simulink model "Hello_World"  (R2014a)
settings: Solver=FixedStepDiscrete  StartTime=0.0  StopTime=10  FixedStep=0.01  RelTol=1e-3
PostLoadFcn:
  | T = 0.1;
CloseFcn:
  | clear T
settings Model: Creator=The MathWorks Inc.  LastModifiedBy=darenlee
settings OptimizationCC: OptimizeModelRefInitCode=on  LifeSpan=1  MaxStackSize=64
settings DebuggingCC: UnderspecifiedInitializationDetection=Classic
settings HardwareCC: ProdLargestAtomicInteger=Long  ProdLargestAtomicFloat=Double  ProdEndianess=LittleEndian  ProdHWDeviceType=ARM Compatible->ARM Cortex
settings RTWCC: SystemTargetFile=ert.tlc  TemplateMakefile=ert_default_tmf  PostCodeGenCommand=; codertarget.postCodeGenHookCommand(h)  Description=Embedded Coder  GenerateReport=on  ProcessScript=ert_make_rtw_hook  Toolchain=Code Sourcery  IncludeHyperlinkInReport=on  LaunchReport=on  GenerateTraceInfo=on  GenerateTraceReport=on  GenerateTraceReportSl=on  GenerateTraceReportSf=on  GenerateTraceReportEml=on
settings CodeAppCC: IgnoreCustomStorageClasses=off
settings ERTTargetCC: ParMdlRefBuildCompliant=on  CompOptLevelCompliant=on  ConcurrentExecutionCompliant=on  ERTFirstTimeCompliant=on  ModelStepFunctionPrototypeControlCompliant=on  CPPClassGenCompliant=on  ExtMode=on  ExtModeMexArgs='192.168.1.1' 1 17725  InlinedParameterPlacement=Hierarchical

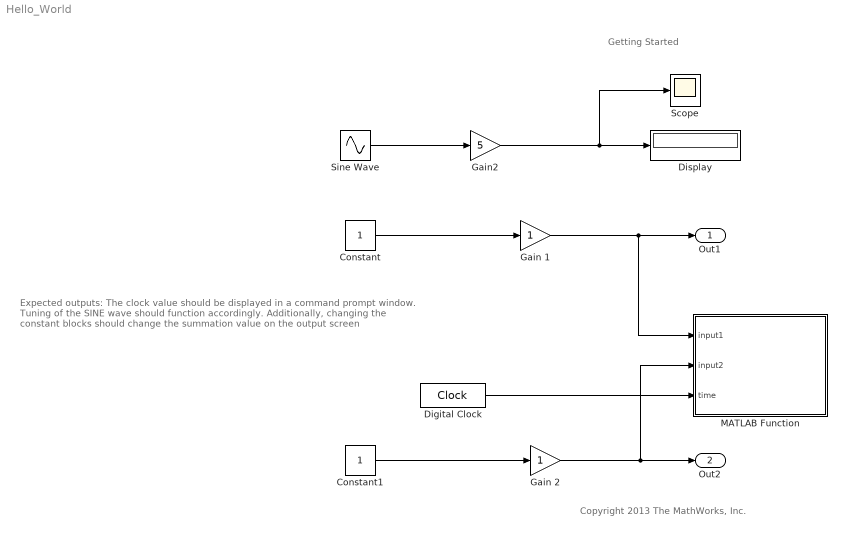
== system Hello_World ==
  note: Expected outputs:
      |
      | The clock value should be displayed in a command prompt window. Tuning
      | of the SINE wave should function accordingly. Additionally, changing the
      | constant blocks should change the summation value on the output screen
  note: Getting Started
  note: Copyright 2013 The MathWorks, Inc.
  Constant : Constant
  Constant1 : Constant
  Digital Clock : DigitalClock  SampleTime=0.1
  Display : Display
  Gain 1 : Gain
  Gain 2 : Gain
  Gain2 : Gain  Gain=5
  MATLAB Function : MATLAB Function  TreatAsAtomicUnit=on
  Scope : Scope
  Sine Wave : Sin  Frequency=1/2  SampleTime=0.01
  Out1 : Outport
  Out2 : Outport  Port=2
  wires:
  Constant/1 -> Gain 1/1
  Gain 1/1 -> MATLAB Function/1(input1), Out1/1
  Constant1/1 -> Gain 2/1
  Gain 2/1 -> MATLAB Function/2(input2), Out2/1
  Digital Clock/1 -> MATLAB Function/3(time)
  Sine Wave/1 -> Gain2/1
  Gain2/1 -> Scope/1, Display/1

== matlab function Hello_World/MATLAB Function ==
  data: input1 input; input2 input; time input
function print_me(input1,input2,time)
%#codegen
sum = input1 + input2;

fmt1 = ['--- The sum of the two inputs is %f --- The current sim time is: %f ' char(10) char(0)];
coder.ceval('printf',coder.rref(fmt1), sum,time);

% coder.ceval('printf','One plus one is: %f |  The sim time is: %f ',sum,time);
% coder.ceval('printf','\n');



end
